simulink model "rb"  (R2025a)
settings: Solver=VariableStepAuto  StartTime=0.0  StopTime=10.0  RelTol=1e-3
undefined symbols (not defined in the file): doppler
libraries: commchan3 x2, commdigbbndpm3 x2, commsink2 x1, commrandsrc3 x1
settings Model: Creator=haris  LastModifiedBy=haris

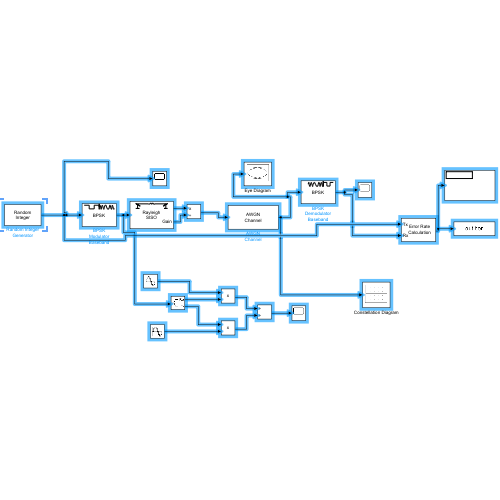
[thumbnail: Simulink's stored preview of the top-level diagram]
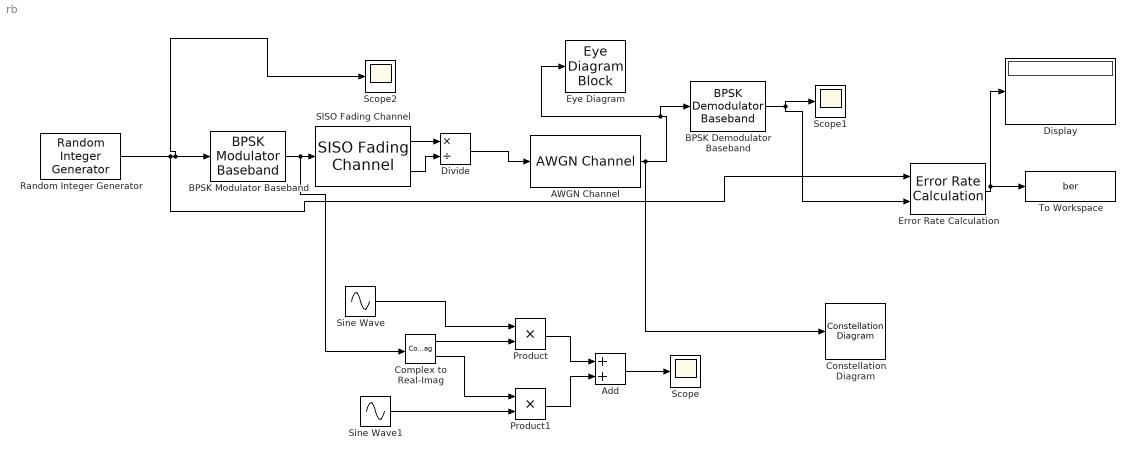
== system rb ==
  AWGN Channel : commchan3/AWGN Channel  LegacyMode=off  NoiseMethod="Signal to noise ratio  (Eb/No)"  noiseMode="Signal to noise ratio  (SNR)"  EbNo=EbNo  EsNo=10  SNR=eb  BitsPerSymbol=1  SignalPower=1  SpecifySymbolPeriod=off  SamplesPerSymbol=1  SymbolPeriod=1  VarianceSource=Parameter  Variance=1  RandomStream=Global stream  Seed=67  SimulateUsing=Code generation
  Add : Sum
  BPSK Demodulator Baseband : commdigbbndpm3/BPSK Demodulator Baseband  DecType=Hard decision  VarSource=Dialog  Variance=1  Ph=0  outDtype=Inherit via internal rule  derotateFactorWordLen=16  derotateFactorDataTypeStr=Inherit: Same word length as input  derotateFactorLastDataTypeStr=Inherit: Same word length as input
  BPSK Modulator Baseband : commdigbbndpm3/BPSK Modulator Baseband  Ph=0  outDtype=double  outWordLen=16  outUDDataType=sfix(16)  outFracLenMode=Best precision  outFracLen=15  outDataTypeStr=double  outLastDataTypeStr=double
  Complex to Real-Imag : ComplexToRealImag
  Constellation Diagram : ConstellationDiagram  WindowPosition=[639.000000,114.000000,600.000000,600.000000,]  ScopeFrameLocation=window
  Display : Display
  Divide : Product  Inputs=*/
  Error Rate Calculation : commsink2/Error Rate Calculation  N=0  st_delay=0  cp_mode=Entire frame  subframe=[]  PMode=Port  WsName=ber  RsMode2=off  stop=off  numErr=100  maxBits=1e6
  Eye Diagram : EyeDiagramBlock  WindowPosition=[368.000000,182.000000,800.000000,500.000000,]  ScopeFrameLocation=window
  Product : Product
  Product1 : Product
  Random Integer Generator : commrandsrc3/Random Integer Generator  SetSize=2  SeedSource=Auto  Seed=0  SampleTime=1  SamplesPerFrame=1000  OutputDataType=double  SimulateUsing=Interpreted execution
  SISO Fading Channel : commchan3/SISO Fading Channel  InheritSampleRate=on  SampleRate=1  PathDelays=0  AveragePathGains=0  NormalizePathGains=on  FadingDistribution=Rayleigh  KFactor=3  DirectPathDopplerShift=0  DirectPathInitialPhase=0  MaximumDopplerShift=0.01  DopplerSpectrum=doppler('Jakes')  RandomStream=mt19937ar with seed  Seed=67  PathGainsOutputPort=on  ChannelFilterDelayOutputPort=off  SimulateUsing=Interpreted execution  Visualization=Off  PathsForDopplerDisplay=1  SamplesToDisplay=25%
  Scope : Scope
      settings: ActiveDisplayYMinimum=-1  ActiveDisplayYMaximum=1
  Scope1 : Scope
      settings: ActiveDisplayYMinimum=-1  ActiveDisplayYMaximum=1
  Scope2 : Scope
      settings: ActiveDisplayYMinimum=-1  ActiveDisplayYMaximum=1  DataLoggingVariableName=ScopeData2
  Sine Wave : Sin  Frequency=8*pi  SampleTime=0.001
  Sine Wave1 : Sin  Frequency=8*pi  Phase=pi/2  SampleTime=0.001
  To Workspace : ToWorkspace  VariableName=ber  SampleTime=-1
      settings: Save2DSignal=2-D array (concatenate along first dimension)
  wires:
  SISO Fading Channel/1 -> Divide/1
  SISO Fading Channel/2 -> Divide/2
  Divide/1 -> AWGN Channel/1
  Product/1 -> Add/1
  BPSK Demodulator Baseband/1 -> Error Rate Calculation/2, Scope1/1
  Add/1 -> Scope/1
  Error Rate Calculation/1 -> To Workspace/1, Display/1
  Sine Wave1/1 -> Product1/2
  Product1/1 -> Add/2
  Sine Wave/1 -> Product/1
  BPSK Modulator Baseband/1 -> Complex to Real-Imag/1, SISO Fading Channel/1
  Random Integer Generator/1 -> BPSK Modulator Baseband/1, Scope2/1, Error Rate Calculation/1
  Complex to Real-Imag/1 -> Product/2
  AWGN Channel/1 -> Constellation Diagram/1, BPSK Demodulator Baseband/1, Eye Diagram/1
  Complex to Real-Imag/2 -> Product1/1
